simulink model "vehicle_dynamics"  (R2024b)
settings: Solver=VariableStepAuto  StartTime=0.0  StopTime=10.0  RelTol=1e-3
libraries: slpidlib x1, simulink x1
settings Model: Creator=shivathmikavadla  LastModifiedBy=shivathmikavadla

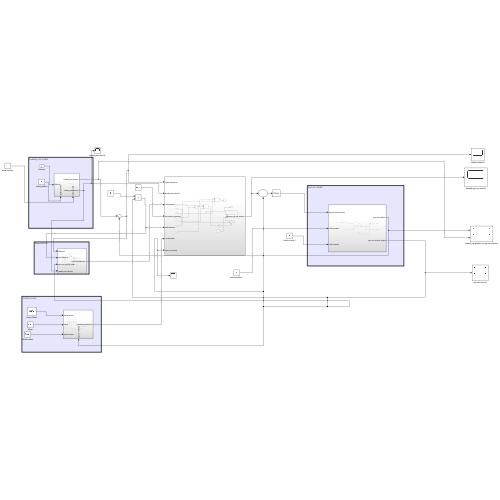
[thumbnail: Simulink's stored preview of the top-level diagram]
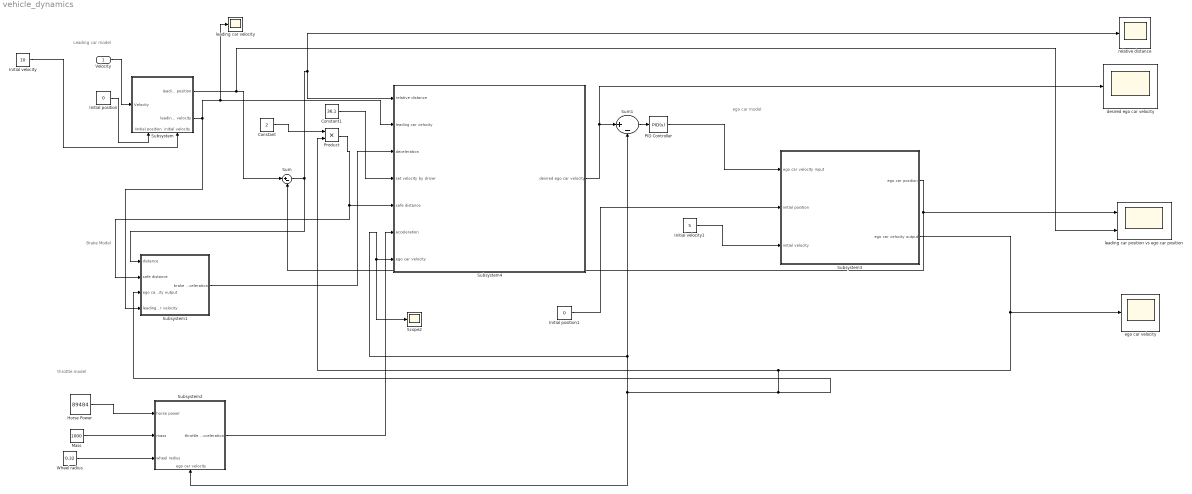
== system vehicle_dynamics ==
  note: ego car model
  note: throttle model
  note: Brake Model
  note: Leading car model
  Velocity : Inport
  Constant : Constant  Value=2
  Constant1 : Constant  Value=36.1
  Horse Power : Constant  Value=89484
  Initial position : Constant  Value=0
  Initial position1 : Constant  Value=0
  Initial velocity : Constant  Value=10
  Initial velocity1 : Constant  Value=5
  Mass : Constant  Value=1000
  PID Controller : slpidlib/PID Controller  Controller=PID  Form=Parallel  TimeDomain=Continuous-time  UseExternalTs=off  SampleTime=-1  IntegratorMethod=Forward Euler  FilterMethod=Forward Euler  ControllerParametersSource=internal  P=1  I=1  UseKiTs=off  D=0  UseExternalDerivativeSource=off  N=100  UseFilter=on  TunerSelectOption=Transfer Function Based (PID Tuner App)  InitialConditionSource=internal  InitialConditionForIntegrator=0  InitialConditionForFilter=0  DifferentiatorICPrevScaledInput=0  ExternalReset=none  TrackingMode=off  Kt=1  LimitOutput=off  SatLimitsSource=internal  UpperSaturationLimit=inf  LowerSaturationLimit=-inf  LinearizeAsGain=on  AntiWindupMode=none  Kb=1  LimitIntegrator=off  UpperIntegratorSaturationLimit=inf  LowerIntegratorSaturationLimit=-inf  POutMin=[]  POutMax=[]  IOutMin=[]  IOutMax=[]  DOutMin=[]  DOutMax=[]  NOutMin=[]  NOutMax=[]  SumOutMin=[]  SumOutMax=[]  SaturationOutMin=[]  SaturationOutMax=[]  PParamMin=[]  PParamMax=[]  IParamMin=[]  IParamMax=[]  DParamMin=[]  DParamMax=[]  NParamMin=[]  NParamMax=[]  KbParamMin=[]  KbParamMax=[]  KtParamMin=[]  KtParamMax=[]  KbOutMin=[]  KbOutMax=[]  KtOutMin=[]  KtOutMax=[]  IntegratorOutMin=[]  IntegratorOutMax=[]  FilterOutMin=[]  FilterOutMax=[]  SumI1OutMin=[]  SumI1OutMax=[]  SumI2OutMin=[]  SumI2OutMax=[]  SumI3OutMin=[]  SumI3OutMax=[]  SumI4OutMin=[]  SumI4OutMax=[]  SumDOutMin=[]  SumDOutMax=[]  DifferentiatorOutMin=[]  DifferentiatorOutMax=[]  FilterDiffOutCoefMin=[]  FilterDiffOutCoefMax=[]  ReciprocalOutMin=[]  ReciprocalOutMax=[]  SumDenOutMin=[]  SumDenOutMax=[]  SumNumOutMin=[]  SumNumOutMax=[]  DivideOutMin=[]  DivideOutMax=[]  UdiffTsProdOutMin=[]  UdiffTsProdOutMax=[]  NTsProdOutMin=[]  NTsProdOutMax=[]  UintegralTsProdOutMin=[]  UintegralTsProdOutMax=[]  UngainTsProdOutMin=[]  UngainTsProdOutMax=[]  ClampingZeroOutDataTypeStr=Inherit: Inherit via back propagation  ClampingZeroOutMin=[]  ClampingZeroOutMax=[]  FilterDenConstantOutDataTypeStr=Inherit: Inherit via back propagation  FilterDenConstantOutMin=[]  FilterDenConstantOutMax=[]  PCopyOutDataTypeStr=Inherit: Inherit via back propagation  PCopyOutMin=[]  PCopyOutMax=[]  NCopyOutDataTypeStr=Inherit: Inherit via back propagation  NCopyOutMin=[]  NCopyOutMax=[]  IntegratorContinuousStateAttributes=''  IntegratorStateMustResolveToSignalObject=off  IntegratorRTWStateStorageClass=Auto  FilterContinuousStateAttributes=''  FilterStateMustResolveToSignalObject=off  FilterRTWStateStorageClass=Auto  ParallelPVariant=InternalParameters  IdealPVariant=Disabled  IVariant=InternalParameters  DVariant=InternalParameters  IntegratorVariant=Continuous  SatVariant=Disabled  AWVariant=Passthrough  PCopyVariant=Disabled  TRVariant=Disabled  FdbkBlocksVariant=Forward  IdealPFdbkVariant=Disabled  SatFdbkVariant=Disabled  DerivativeFilterVariant=ContFilter  NVariant=InternalParameters  NCopyVariant=Disabled  FilterICVariant=InternalICsFilter  IntegratorICVariant=InternalICs  ExternalResetVariant=Disabled  TRSumVariant=Passthrough  SumFdbkVariant=Disabled  SumVariant=Sum_PID  TsampFilterVariant=InternalTs  TsampNgainVariant=Passthrough  TsampIntegralVariant=Disabled_SignalSpec  ExternalSaturationOutDataTypeStr=Inherit: Same as second input  DerivativeSourceVariant=ErrorSignal  PreIntVariant=InternalPreInt
  Product : Product
  Scope2 : Scope
  Subsystem : Subsystem
      settings: PortSchema="{\"entries\":[{\"content\":{\"sides\":[{\"content\":{\"connectorIds\":[\"In1\"]},\"type\":\"ConnectorPlacement.EquallySpacedRectSide\",\"uuid\":\"88e62f58-abb7-424e-bece-cb0affe26b20\"},{\"content\":{\"connectorIds\":[\"Out1\",\"Out2\"],\"side\":\"RIGHT\"},\"type\":\"ConnectorPlacement.EquallySpacedRectSide\",\"uuid\":\"86853464-5600-4523-8146-b34d4afbe922\"},{\"content\":{\"side\":\"TOP\"},\"type\":\"ConnectorPlacement.EquallySpacedRectSide\",\"uuid\":\"e94ff8c3-f3cd-4fad-ad77-705efd5e2c66\"},{\"content\":{\"connectorIds\":[\"In2\",\"In3\"],\"side\":\"BOTTOM\"},\"type\":\"ConnectorPlacement.EquallySpacedRectSide\",\"uuid\":\"327904ee-22ab-44ca-b63a-b33e6d8501f5\"}]},\"type\":\"ConnectorPlacement.EquallySpacedConnector\",\"uuid\":\"b5b9b1e1-879b-406c-a2bb-6c59d1b88566\"}],\"packageUris\":[\"http://schema.mathworks.com/mf0/Connector/R2020b\"],\"version\":\"1.0\"}"
  Subsystem1 : Subsystem
  Subsystem2 : Subsystem
      settings: PortSchema="{\"entries\":[{\"content\":{\"sides\":[{\"content\":{\"connectorIds\":[\"In1\",\"In2\",\"In3\"]},\"type\":\"ConnectorPlacement.EquallySpacedRectSide\",\"uuid\":\"6f7fc6ef-cf55-43d9-98d6-98847b3edffa\"},{\"content\":{\"connectorIds\":[\"Out1\"],\"side\":\"RIGHT\"},\"type\":\"ConnectorPlacement.EquallySpacedRectSide\",\"uuid\":\"51f9bcc9-e8b5-40a1-8c1e-180b9cd97441\"},{\"content\":{\"side\":\"TOP\"},\"type\":\"ConnectorPlacement.EquallySpacedRectSide\",\"uuid\":\"e97a63e6-5654-42c9-b5c3-f805b12ccfeb\"},{\"content\":{\"connectorIds\":[\"In4\"],\"side\":\"BOTTOM\"},\"type\":\"ConnectorPlacement.EquallySpacedRectSide\",\"uuid\":\"2824cb99-de13-4057-9f89-027cc5106a03\"}]},\"type\":\"ConnectorPlacement.EquallySpacedConnector\",\"uuid\":\"a5bbedff-455e-4eaa-9ca7-282e30a1540b\"}],\"packageUris\":[\"http://schema.mathworks.com/mf0/Connector/R2020b\"],\"version\":\"1.0\"}"
  Subsystem3 : Subsystem
  Subsystem4 : Subsystem
  Sum : Sum  Inputs=|+-
  Sum1 : Sum  Inputs=|+-
  Wheel radius : Constant  Value=0.32
  desired ego car velocity : Scope
  ego car velocity : Scope
  leading car position vs ego car position : Scope  NumInputPorts=2
  leading car velocity : Scope
  relative distance : Scope
  wires:
  Velocity/1 -> Subsystem/1(Velocity)
  Initial position/1 -> Subsystem/2(Iinitial position)
  Initial velocity/1 -> Subsystem/3(initial velocity)
  Subsystem/2(leading car velocity) -> leading car velocity/1, Subsystem4/2(leading car velocity), Subsystem1/4(leading car velocity)
  Horse Power/1 -> Subsystem2/1(horse power)
  Mass/1 -> Subsystem2/2(mass)
  Wheel radius/1 -> Subsystem2/3(wheel radius)
  Subsystem/1(leading car position) -> leading car position vs ego car position/2, Sum/1
  Sum1/1 -> PID Controller/1
  Subsystem3/2(ego car velocity output) -> Product/2, Subsystem2/4(ego car velocity), Sum1/2, Scope2/1, Subsystem4/7(ego car velocity), Subsystem1/3(ego car velocity output), ego car velocity/1
  Subsystem3/1(ego car position) -> Sum/2, leading car position vs ego car position/1
  Sum/1 -> Subsystem4/1(relative distance), relative distance/1, Subsystem1/1(distance)
  Subsystem1/1(brake deceleration) -> Subsystem4/3(" deceleration")
  Subsystem2/1(throttle acceleration) -> Subsystem4/6(" acceleration")
  Constant/1 -> Product/1
  Initial position1/1 -> Subsystem3/2(initial position)
  Initial velocity1/1 -> Subsystem3/3(initial velocity)
  Product/1 -> Subsystem1/2(safe distance), Subsystem4/5(safe distance)
  Constant1/1 -> Subsystem4/4(set velocity by driver)
  Subsystem4/1(desired ego car velocity) -> desired ego car velocity/1, Sum1/1
  PID Controller/1 -> Subsystem3/1(ego car velocity input)

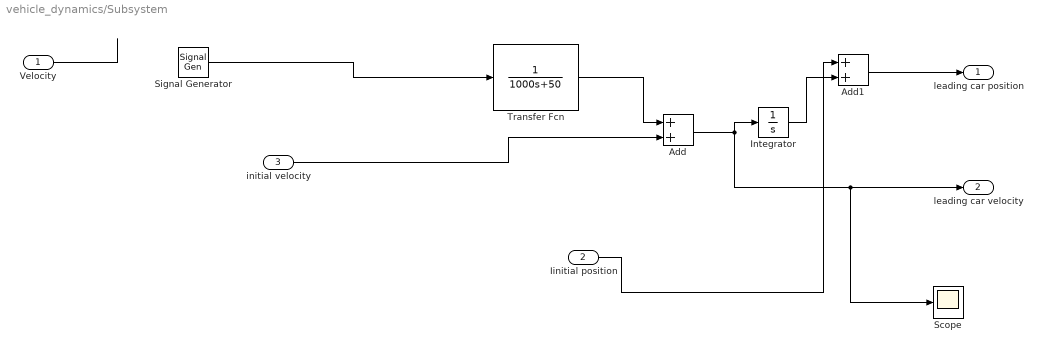
== system vehicle_dynamics/Subsystem ==
  Velocity : Inport
  Iinitial position : Inport  Port=2
  initial velocity : Inport  Port=3
  Add : Sum
  Add1 : Sum
  Integrator : Integrator
  Scope : Scope
  Signal Generator : SignalGenerator  Units=rad/sec
  Transfer Fcn : TransferFcn  Denominator=[1000 50]
  leading car position : Outport
  leading car velocity : Outport  Port=2
  wires:
  Transfer Fcn/1 -> Add/1
  initial velocity/1 -> Add/2
  Iinitial position/1 -> Add1/1
  Add/1 -> Scope/1, leading car velocity/1, Integrator/1
  Integrator/1 -> Add1/2
  Add1/1 -> leading car position/1
  Velocity/1 -> ?
  Signal Generator/1 -> Transfer Fcn/1

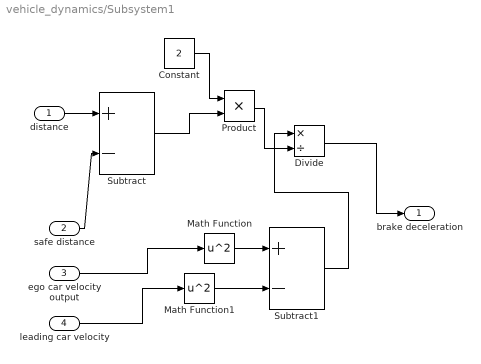
== system vehicle_dynamics/Subsystem1 ==
  distance : Inport
  safe distance : Inport  Port=2
  ego car velocity output : Inport  Port=3
  leading car velocity : Inport  Port=4
  Constant : Constant  Value=2
  Divide : Product  Inputs=*/
  Math Function : Math  Operator=square
  Math Function1 : Math  Operator=square
  Product : Product
  Subtract : Sum  Inputs=+-
  Subtract1 : Sum  Inputs=+-
  brake deceleration : Outport
  wires:
  distance/1 -> Subtract/1
  safe distance/1 -> Subtract/2
  ego car velocity output/1 -> Math Function/1
  leading car velocity/1 -> Math Function1/1
  Math Function/1 -> Subtract1/1
  Math Function1/1 -> Subtract1/2
  Constant/1 -> Product/1
  Subtract/1 -> Product/2
  Subtract1/1 -> Divide/1
  Product/1 -> Divide/2
  Divide/1 -> brake deceleration/1

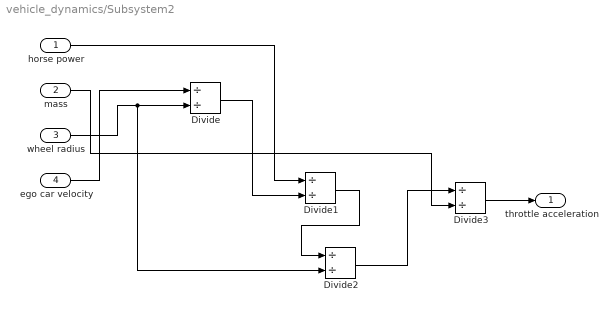
== system vehicle_dynamics/Subsystem2 ==
  horse power : Inport
  mass : Inport  Port=2
  wheel radius : Inport  Port=3
  ego car velocity : Inport  Port=4
  Divide{,1..3} (4 alike) : Product  Inputs=//
  throttle acceleration : Outport
  wires:
  horse power/1 -> Divide1/1
  ego car velocity/1 -> Divide/1
  wheel radius/1 -> Divide2/2, Divide/2
  Divide/1 -> Divide1/2
  Divide1/1 -> Divide2/1
  Divide2/1 -> Divide3/1
  mass/1 -> Divide3/2
  Divide3/1 -> throttle acceleration/1

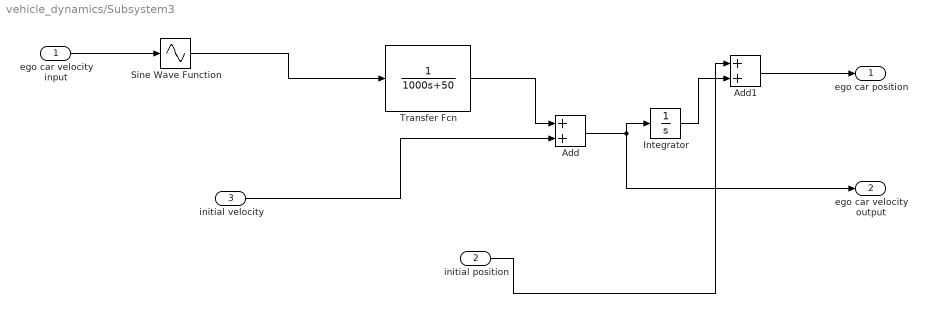
== system vehicle_dynamics/Subsystem3 ==
  ego car velocity input : Inport
  initial position : Inport  Port=2
  initial velocity : Inport  Port=3
  Add : Sum
  Add1 : Sum
  Integrator : Integrator
  Sine Wave Function : Sin  TimeSource=Use external signal  SampleTime=0
  Transfer Fcn : TransferFcn  Denominator=[1000 50]
  ego car position : Outport
  ego car velocity output : Outport  Port=2
  wires:
  Integrator/1 -> Add1/2
  Transfer Fcn/1 -> Add/1
  initial position/1 -> Add1/1
  initial velocity/1 -> Add/2
  Add/1 -> ego car velocity output/1, Integrator/1
  Add1/1 -> ego car position/1
  ego car velocity input/1 -> Sine Wave Function/1
  Sine Wave Function/1 -> Transfer Fcn/1

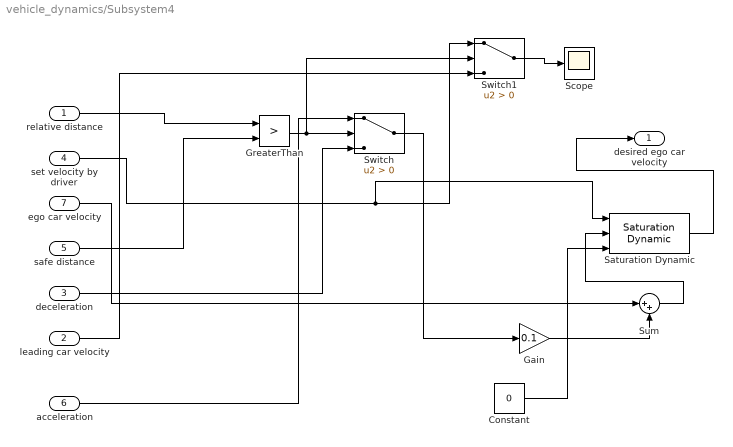
== system vehicle_dynamics/Subsystem4 ==
  relative distance : Inport
  leading car velocity : Inport  Port=2
  " deceleration" : Inport  Port=3
  set velocity by driver : Inport  Port=4
  safe distance : Inport  Port=5
  " acceleration" : Inport  Port=6
  ego car velocity : Inport  Port=7
  Constant : Constant  Value=0
  Gain : Gain  Gain=0.1
  GreaterThan : RelationalOperator  Operator=>  OutDataTypeStr=boolean  RndMeth=Simplest  InputSameDT=off
  Saturation Dynamic : simulink/Discontinuities/Saturation Dynamic  OutMin=[]  OutMax=[]  OutDataTypeStr=Inherit: Same as second input  OutDataType=fixdt(1, 16)  OutScaling=2^-10  DoSatur=off
  Scope : Scope
  Sum : Sum  Inputs=|++
  Switch : Switch  Criteria=u2 > Threshold  SaturateOnIntegerOverflow=off  InputSameDT=off
  Switch1 : Switch  Criteria=u2 > Threshold  SaturateOnIntegerOverflow=off  InputSameDT=off
  desired ego car velocity : Outport
  wires:
  safe distance/1 -> GreaterThan/2
  relative distance/1 -> GreaterThan/1
  GreaterThan/1 -> Switch1/2, Switch/2
  " acceleration"/1 -> Switch/1
  " deceleration"/1 -> Switch/3
  set velocity by driver/1 -> Saturation Dynamic/1, Switch1/1
  leading car velocity/1 -> Switch1/3
  Switch/1 -> Gain/1
  Gain/1 -> Sum/2
  ego car velocity/1 -> Sum/1
  Sum/1 -> Saturation Dynamic/2
  Constant/1 -> Saturation Dynamic/3
  Saturation Dynamic/1 -> desired ego car velocity/1
  Switch1/1 -> Scope/1
